simulink model "pipeline_discrete_pid"  (R2023a)
settings: Solver=ode45  StartTime=0.0  StopTime=200  MaxStep=0.01  RelTol=1e-3
settings Model: Creator=Theodora  LastModifiedBy=Theodora

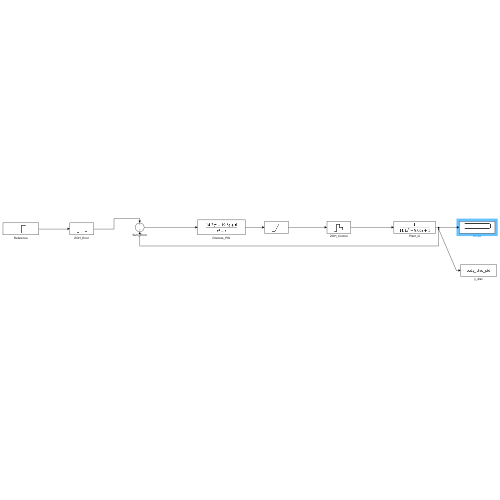
[thumbnail: Simulink's stored preview of the top-level diagram]
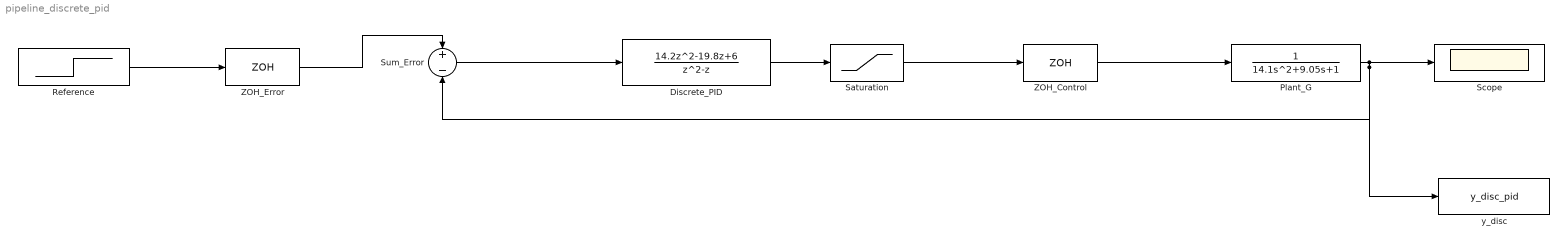
== system pipeline_discrete_pid ==
  Discrete_PID : DiscreteTransferFcn  Numerator=[14.2 -19.8 6]  Denominator=[1 -1 0]  SampleTime=1
  Plant_G : TransferFcn  Numerator=1  Denominator=[14.1 9.05 1]
  Reference : Step  Time=0  SampleTime=0
  Saturation : Saturate  UpperLimit=2  LowerLimit=0
  Scope : Scope
  Sum_Error : Sum  Inputs=+-
  ZOH_Control : ZeroOrderHold
  ZOH_Error : ZeroOrderHold
  y_disc : ToWorkspace  VariableName=y_disc_pid  SampleTime=-1
  wires:
  Plant_G/1 -> Sum_Error/2, y_disc/1, Scope/1
  Sum_Error/1 -> Discrete_PID/1
  Discrete_PID/1 -> Saturation/1
  Saturation/1 -> ZOH_Control/1
  ZOH_Control/1 -> Plant_G/1
  Reference/1 -> ZOH_Error/1
  ZOH_Error/1 -> Sum_Error/1
